simulink model "DMC_discrete_system"  (R2016a)
settings: Solver=VariableStepAuto  StartTime=0.0  StopTime=10.0  RelTol=1e-3
values from neighbouring files (symbols this model uses):
  a = step(sys,T:T:N*T)    [DMC_Zheng.m]    (also in z3.m)
  C_2 = zeros(1,N);C_2(1) = 1    [z3.m]
  d = C*inv(A'*Q*A+R)*A'*Q    [DMC_Zheng.m]    (also in z3.m)
  h = ones(N,1)    [DMC_Zheng.m]    (also in z3.m = 1*ones(N,1))
  I = [I_1,I_2]    [DMC_Zheng.m]    (also in z3.m)
  S = zeros(N,N)    [DMC_Zheng.m]    (also in z3.m)
  T = 0.01    [DMC_Zheng.m]    (also in z3.m)
undefined symbols (not defined in the file or in its folder): den1, num1
settings Model: Creator=政  LastModifiedBy=政

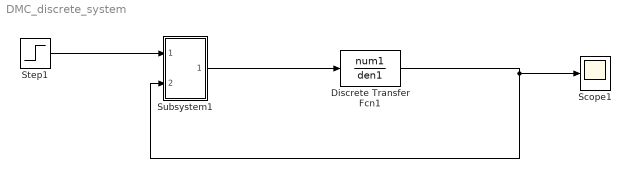
== system DMC_discrete_system ==
  Discrete Transfer Fcn1 : DiscreteTransferFcn  Numerator=num1  Denominator=den1
  Scope1 : Scope
  Step1 : Step  Time=0  SampleTime=T
  Subsystem1 : Subsystem
  wires:
  Step1/1 -> Subsystem1/1(In1)
  Discrete Transfer Fcn1/1 -> Subsystem1/2(In2), Scope1/1
  Subsystem1/1(Out1) -> Discrete Transfer Fcn1/1

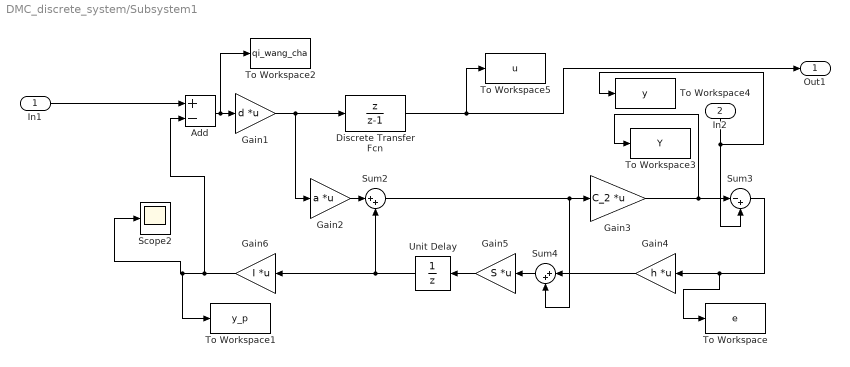
== system DMC_discrete_system/Subsystem1 ==
  In1 : Inport
  In2 : Inport  Port=2
  Add : Sum  Inputs=+-
  Discrete Transfer Fcn : DiscreteTransferFcn  Numerator=[1 0]  Denominator=[1 -1]
  Gain1 : Gain  Gain=d  Multiplication=Matrix(K*u)
  Gain2 : Gain  Gain=a  Multiplication=Matrix(K*u)
  Gain3 : Gain  Gain=C_2  Multiplication=Matrix(K*u)
  Gain4 : Gain  Gain=h  Multiplication=Matrix(K*u)
  Gain5 : Gain  Gain=S  Multiplication=Matrix(K*u)
  Gain6 : Gain  Gain=I  Multiplication=Matrix(K*u)
  Scope2 : Scope
  Sum2 : Sum  Inputs=|++
  Sum3 : Sum  Inputs=|-+
  Sum4 : Sum  Inputs=|++
  To Workspace : ToWorkspace  VariableName=e  SaveFormat=Timeseries  SampleTime=-1
  To Workspace1 : ToWorkspace  VariableName=y_p  SaveFormat=Timeseries  SampleTime=-1
  To Workspace2 : ToWorkspace  VariableName=qi_wang_cha  SaveFormat=Timeseries  SampleTime=-1
  To Workspace3 : ToWorkspace  VariableName=Y  SaveFormat=Timeseries  SampleTime=-1
  To Workspace4 : ToWorkspace  VariableName=y  SaveFormat=Timeseries  SampleTime=-1
  To Workspace5 : ToWorkspace  VariableName=u  SaveFormat=Timeseries  SampleTime=-1
  Unit Delay : UnitDelay  SampleTime=-1
  Out1 : Outport
  wires:
  Gain3/1 -> To Workspace3/1, Sum3/1
  Add/1 -> To Workspace2/1, Gain1/1
  Gain1/1 -> Gain2/1, Discrete Transfer Fcn/1
  Gain2/1 -> Sum2/1
  Sum2/1 -> Sum4/2, Gain3/1
  In1/1 -> Add/1
  Sum4/1 -> Gain5/1
  Gain5/1 -> Unit Delay/1
  Unit Delay/1 -> Sum2/2, Gain6/1
  Gain4/1 -> Sum4/1
  Gain6/1 -> Add/2, To Workspace1/1, Scope2/1
  Sum3/1 -> To Workspace/1, Gain4/1
  In2/1 -> To Workspace4/1, Sum3/2
  Discrete Transfer Fcn/1 -> To Workspace5/1, Out1/1
